simulink model "Par_model_sim_CHBjt9"  (R2023b)
settings: Solver=FixedStepAuto  StartTime=0.0  StopTime=5  FixedStep=1e-6  RelTol=1e-3
InitFcn:
  | sysinit
values from neighbouring files (symbols this model uses):
  C = 0.0234    [sysinit.m]
  f = 50    [sysinit.m]
  f_out = frequency_out_start : frequency_out_interval : frequency_out_end    [simout_chb_par.m]    (also in simout_chbjt_par.m = frequency_modulate_start : frequency_modulate_interval : fre)
  fn = 50    [sysinit.m]
  L = 0.002    [sysinit.m]
  L_ori = 0.02    [sysinit.m]
  L_sec = 0.06    [sysinit.m]
  m = 0.95    [sysinit.m]
  P0 = 8e6    (= 8000000)    [sysinit.m]
  R = 1.5    [sysinit.m]
  Source_Amp = 10000    [sysinit.m]
  st = 1e-6    (= 1e-06)    [sysinit.m]
  Td = 15e-7    (= 1.5e-06)    [sysinit.m]
  Ts2 = 0.5e-3    (= 0.0005)    [sysinit.m]
  U_dcN = 2500    [sysinit.m]
  Ul_in = 1900    [sysinit.m]
undefined symbols (not defined in the file or in its folder): magnitude
libraries: spsSeriesRLCBranchLib x123, spsDiodeLib x60, spsIGBTLib x48, spsMeanLib x20, spsCurrentMeasurementLib x16, spsThreePhaseVIMeasurementLib x13, spsOnDelayLib x12, spsUniversalBridgeLib x12, spsMultiWindingTransformerLib x9, simulink x5, spsRMSLib x4, spsVoltageMeasurementLib x3
(part 1 of 3)
settings Model: SimulationMode=accelerator  Creator=Jhchen  LastModifiedBy=Jhchen
settings DataIOCC: ReturnWorkspaceOutputs=off
settings DebuggingCC: RTPrefix=warning

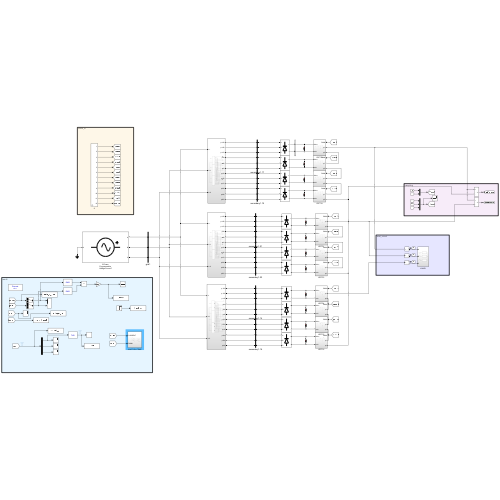
[thumbnail: Simulink's stored preview of the top-level diagram]
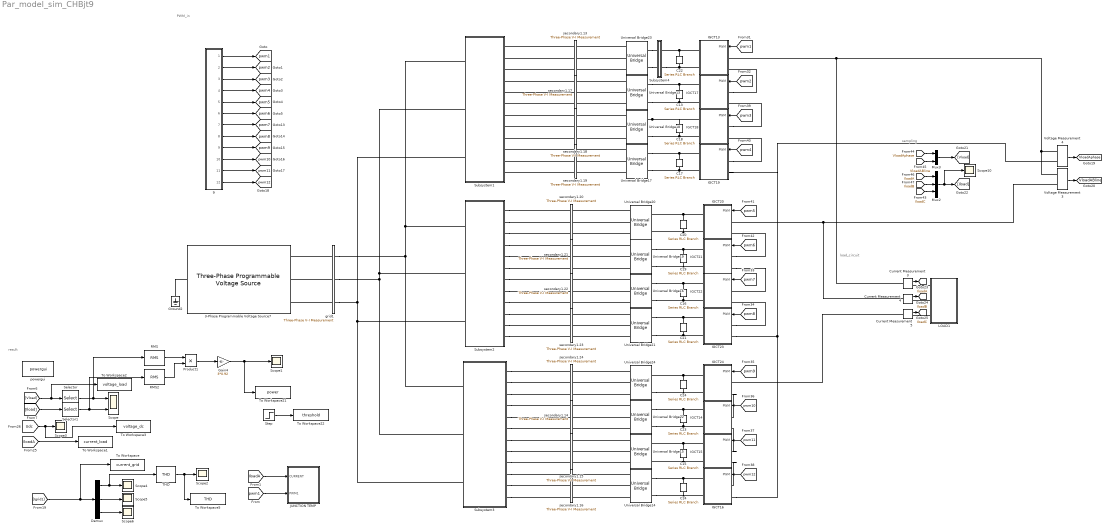
== system Par_model_sim_CHBjt9 ==
  note: PWM_in
  note: result
  note: load_circuit
  note: sampling
  3-Phase Programmable Voltage Source7 : spsThreePhaseProgrammableVoltageSourceLib/Three-Phase Programmable Voltage Source  PositiveSequence=[Source_Amp 0 fn]  VariationEntity=None  VariationType=Step  VariationTypeAlt=Step  VariationStep=0.5  VariationRate=10  VariationMagnitude=0.3  VariationFrequency=2  VariationTiming=[0.05 1]  VariationPhaseA=off  Amplitudes=[1 0.8 1.2 1.0]  TimeValues=[0 0.1 0.15 0.2]  HarmonicGeneration=off  HarmonicA=[5 0.08 -45 2]  HarmonicB=[2 0 0 2]  Timing="[0.1  1]"  BusType=swing  Pref=0  Qref=0  Qmin=-inf  Qmax=inf
  9 : Subsystem  mask{m=m, f=f, f_car=f_out, tt=1/8, ttd=Td}
      mask prompts: m "m_p"; f "f_module"; f_car "f_carrier"; tt "ts"; ttd "td"
      mask DialogControl ParameterGroupVar Prompt: 参数
  C{13..24} (12 alike) : spsSeriesRLCBranchLib/Series RLC Branch  LConnTagsString=__new0  RConnTagsString=__new0  BranchType=C  Resistance=0.0001  Inductance=1.0  SetiL0=off  InitialCurrent=0  Capacitance=C  Setx0=on  InitialVoltage=2500  Measurements=None
  Current Measurement3 : spsCurrentMeasurementLib/Current Measurement  PhasorSimulation=off  OutputType=Complex  PSBequivalent=0
  Current Measurement4 : spsCurrentMeasurementLib/Current Measurement  PhasorSimulation=off  OutputType=Complex  PSBequivalent=0
  Current Measurement5 : spsCurrentMeasurementLib/Current Measurement  PhasorSimulation=off  OutputType=Complex  PSBequivalent=0
  Demux : Demux  Outputs=3
  Gain4 : Gain  Gain=3*0.92
  Ground2 : spsGroundLib/Ground  LConnTagsString=a
  IGCT13 : Subsystem
      settings: PortSchema="{\"entries\":[{\"content\":{\"sides\":[{\"content\":{\"connectorIds\":[\"LConn1\",\"LConn2\"]},\"type\":\"ConnectorPlacement.EquallySpacedRectSide\",\"uuid\":\"3b5227fd-32cc-4097-9a6a-2909540651e9\"},{\"content\":{\"connectorIds\":[\"In1\",\"RConn1\",\"RConn2\"],\"side\":\"RIGHT\"},\"type\":\"ConnectorPlacement.EquallySpacedRectSide\",\"uuid\":\"b0068562-9d9a-456b-acd2-db870c5bcace\"},{\"content\":{\"side\":\"TOP\"},\"type\":\"ConnectorPlacement.EquallySpacedRectSide\",\"uuid\":\"bbecbe08-a8e7-4703-9f6f-443f87d924da\"}]},\"type\":\"ConnectorPlacement.EquallySpacedConnector\",\"uuid\":\"6ec83c7b-e3bb-4502-bc8f-4da9ff103a20\"}],\"packageUris\":[\"http://schema.mathworks.com/mf0/Connector/R2020b\"],\"version\":\"1.0\"}"
  IGCT14 : Subsystem
      settings: PortSchema="{\"entries\":[{\"content\":{\"sides\":[{\"content\":{\"connectorIds\":[\"LConn1\",\"LConn2\"]},\"type\":\"ConnectorPlacement.EquallySpacedRectSide\",\"uuid\":\"3b5227fd-32cc-4097-9a6a-2909540651e9\"},{\"content\":{\"connectorIds\":[\"In1\",\"RConn1\",\"RConn2\"],\"side\":\"RIGHT\"},\"type\":\"ConnectorPlacement.EquallySpacedRectSide\",\"uuid\":\"b0068562-9d9a-456b-acd2-db870c5bcace\"},{\"content\":{\"side\":\"TOP\"},\"type\":\"ConnectorPlacement.EquallySpacedRectSide\",\"uuid\":\"bbecbe08-a8e7-4703-9f6f-443f87d924da\"}]},\"type\":\"ConnectorPlacement.EquallySpacedConnector\",\"uuid\":\"6ec83c7b-e3bb-4502-bc8f-4da9ff103a20\"}],\"packageUris\":[\"http://schema.mathworks.com/mf0/Connector/R2020b\"],\"version\":\"1.0\"}"
  IGCT15 : Subsystem
      settings: PortSchema="{\"entries\":[{\"content\":{\"sides\":[{\"content\":{\"connectorIds\":[\"LConn1\",\"LConn2\"]},\"type\":\"ConnectorPlacement.EquallySpacedRectSide\",\"uuid\":\"3b5227fd-32cc-4097-9a6a-2909540651e9\"},{\"content\":{\"connectorIds\":[\"In1\",\"RConn1\",\"RConn2\"],\"side\":\"RIGHT\"},\"type\":\"ConnectorPlacement.EquallySpacedRectSide\",\"uuid\":\"b0068562-9d9a-456b-acd2-db870c5bcace\"},{\"content\":{\"side\":\"TOP\"},\"type\":\"ConnectorPlacement.EquallySpacedRectSide\",\"uuid\":\"bbecbe08-a8e7-4703-9f6f-443f87d924da\"}]},\"type\":\"ConnectorPlacement.EquallySpacedConnector\",\"uuid\":\"6ec83c7b-e3bb-4502-bc8f-4da9ff103a20\"}],\"packageUris\":[\"http://schema.mathworks.com/mf0/Connector/R2020b\"],\"version\":\"1.0\"}"
  IGCT16 : Subsystem
      settings: PortSchema="{\"entries\":[{\"content\":{\"sides\":[{\"content\":{\"connectorIds\":[\"LConn1\",\"LConn2\"]},\"type\":\"ConnectorPlacement.EquallySpacedRectSide\",\"uuid\":\"3b5227fd-32cc-4097-9a6a-2909540651e9\"},{\"content\":{\"connectorIds\":[\"In1\",\"RConn1\",\"RConn2\"],\"side\":\"RIGHT\"},\"type\":\"ConnectorPlacement.EquallySpacedRectSide\",\"uuid\":\"b0068562-9d9a-456b-acd2-db870c5bcace\"},{\"content\":{\"side\":\"TOP\"},\"type\":\"ConnectorPlacement.EquallySpacedRectSide\",\"uuid\":\"bbecbe08-a8e7-4703-9f6f-443f87d924da\"}]},\"type\":\"ConnectorPlacement.EquallySpacedConnector\",\"uuid\":\"6ec83c7b-e3bb-4502-bc8f-4da9ff103a20\"}],\"packageUris\":[\"http://schema.mathworks.com/mf0/Connector/R2020b\"],\"version\":\"1.0\"}"
  IGCT17 : Subsystem
      settings: PortSchema="{\"entries\":[{\"content\":{\"sides\":[{\"content\":{\"connectorIds\":[\"LConn1\",\"LConn2\"]},\"type\":\"ConnectorPlacement.EquallySpacedRectSide\",\"uuid\":\"3b5227fd-32cc-4097-9a6a-2909540651e9\"},{\"content\":{\"connectorIds\":[\"In1\",\"RConn1\",\"RConn2\"],\"side\":\"RIGHT\"},\"type\":\"ConnectorPlacement.EquallySpacedRectSide\",\"uuid\":\"b0068562-9d9a-456b-acd2-db870c5bcace\"},{\"content\":{\"side\":\"TOP\"},\"type\":\"ConnectorPlacement.EquallySpacedRectSide\",\"uuid\":\"bbecbe08-a8e7-4703-9f6f-443f87d924da\"}]},\"type\":\"ConnectorPlacement.EquallySpacedConnector\",\"uuid\":\"6ec83c7b-e3bb-4502-bc8f-4da9ff103a20\"}],\"packageUris\":[\"http://schema.mathworks.com/mf0/Connector/R2020b\"],\"version\":\"1.0\"}"
  IGCT18 : Subsystem
      settings: PortSchema="{\"entries\":[{\"content\":{\"sides\":[{\"content\":{\"connectorIds\":[\"LConn1\",\"LConn2\"]},\"type\":\"ConnectorPlacement.EquallySpacedRectSide\",\"uuid\":\"3b5227fd-32cc-4097-9a6a-2909540651e9\"},{\"content\":{\"connectorIds\":[\"In1\",\"RConn1\",\"RConn2\"],\"side\":\"RIGHT\"},\"type\":\"ConnectorPlacement.EquallySpacedRectSide\",\"uuid\":\"b0068562-9d9a-456b-acd2-db870c5bcace\"},{\"content\":{\"side\":\"TOP\"},\"type\":\"ConnectorPlacement.EquallySpacedRectSide\",\"uuid\":\"bbecbe08-a8e7-4703-9f6f-443f87d924da\"}]},\"type\":\"ConnectorPlacement.EquallySpacedConnector\",\"uuid\":\"6ec83c7b-e3bb-4502-bc8f-4da9ff103a20\"}],\"packageUris\":[\"http://schema.mathworks.com/mf0/Connector/R2020b\"],\"version\":\"1.0\"}"
  IGCT19 : Subsystem
      settings: PortSchema="{\"entries\":[{\"content\":{\"sides\":[{\"content\":{\"connectorIds\":[\"LConn1\",\"LConn2\"]},\"type\":\"ConnectorPlacement.EquallySpacedRectSide\",\"uuid\":\"3b5227fd-32cc-4097-9a6a-2909540651e9\"},{\"content\":{\"connectorIds\":[\"In1\",\"RConn1\",\"RConn2\"],\"side\":\"RIGHT\"},\"type\":\"ConnectorPlacement.EquallySpacedRectSide\",\"uuid\":\"b0068562-9d9a-456b-acd2-db870c5bcace\"},{\"content\":{\"side\":\"TOP\"},\"type\":\"ConnectorPlacement.EquallySpacedRectSide\",\"uuid\":\"bbecbe08-a8e7-4703-9f6f-443f87d924da\"}]},\"type\":\"ConnectorPlacement.EquallySpacedConnector\",\"uuid\":\"6ec83c7b-e3bb-4502-bc8f-4da9ff103a20\"}],\"packageUris\":[\"http://schema.mathworks.com/mf0/Connector/R2020b\"],\"version\":\"1.0\"}"
  IGCT20 : Subsystem
      settings: PortSchema="{\"entries\":[{\"content\":{\"sides\":[{\"content\":{\"connectorIds\":[\"LConn1\",\"LConn2\"]},\"type\":\"ConnectorPlacement.EquallySpacedRectSide\",\"uuid\":\"3b5227fd-32cc-4097-9a6a-2909540651e9\"},{\"content\":{\"connectorIds\":[\"In1\",\"RConn1\",\"RConn2\"],\"side\":\"RIGHT\"},\"type\":\"ConnectorPlacement.EquallySpacedRectSide\",\"uuid\":\"b0068562-9d9a-456b-acd2-db870c5bcace\"},{\"content\":{\"side\":\"TOP\"},\"type\":\"ConnectorPlacement.EquallySpacedRectSide\",\"uuid\":\"bbecbe08-a8e7-4703-9f6f-443f87d924da\"}]},\"type\":\"ConnectorPlacement.EquallySpacedConnector\",\"uuid\":\"6ec83c7b-e3bb-4502-bc8f-4da9ff103a20\"}],\"packageUris\":[\"http://schema.mathworks.com/mf0/Connector/R2020b\"],\"version\":\"1.0\"}"
  IGCT21 : Subsystem
      settings: PortSchema="{\"entries\":[{\"content\":{\"sides\":[{\"content\":{\"connectorIds\":[\"LConn1\",\"LConn2\"]},\"type\":\"ConnectorPlacement.EquallySpacedRectSide\",\"uuid\":\"3b5227fd-32cc-4097-9a6a-2909540651e9\"},{\"content\":{\"connectorIds\":[\"In1\",\"RConn1\",\"RConn2\"],\"side\":\"RIGHT\"},\"type\":\"ConnectorPlacement.EquallySpacedRectSide\",\"uuid\":\"b0068562-9d9a-456b-acd2-db870c5bcace\"},{\"content\":{\"side\":\"TOP\"},\"type\":\"ConnectorPlacement.EquallySpacedRectSide\",\"uuid\":\"bbecbe08-a8e7-4703-9f6f-443f87d924da\"}]},\"type\":\"ConnectorPlacement.EquallySpacedConnector\",\"uuid\":\"6ec83c7b-e3bb-4502-bc8f-4da9ff103a20\"}],\"packageUris\":[\"http://schema.mathworks.com/mf0/Connector/R2020b\"],\"version\":\"1.0\"}"
  IGCT22 : Subsystem
      settings: PortSchema="{\"entries\":[{\"content\":{\"sides\":[{\"content\":{\"connectorIds\":[\"LConn1\",\"LConn2\"]},\"type\":\"ConnectorPlacement.EquallySpacedRectSide\",\"uuid\":\"3b5227fd-32cc-4097-9a6a-2909540651e9\"},{\"content\":{\"connectorIds\":[\"In1\",\"RConn1\",\"RConn2\"],\"side\":\"RIGHT\"},\"type\":\"ConnectorPlacement.EquallySpacedRectSide\",\"uuid\":\"b0068562-9d9a-456b-acd2-db870c5bcace\"},{\"content\":{\"side\":\"TOP\"},\"type\":\"ConnectorPlacement.EquallySpacedRectSide\",\"uuid\":\"bbecbe08-a8e7-4703-9f6f-443f87d924da\"}]},\"type\":\"ConnectorPlacement.EquallySpacedConnector\",\"uuid\":\"6ec83c7b-e3bb-4502-bc8f-4da9ff103a20\"}],\"packageUris\":[\"http://schema.mathworks.com/mf0/Connector/R2020b\"],\"version\":\"1.0\"}"
  IGCT23 : Subsystem
      settings: PortSchema="{\"entries\":[{\"content\":{\"sides\":[{\"content\":{\"connectorIds\":[\"LConn1\",\"LConn2\"]},\"type\":\"ConnectorPlacement.EquallySpacedRectSide\",\"uuid\":\"3b5227fd-32cc-4097-9a6a-2909540651e9\"},{\"content\":{\"connectorIds\":[\"In1\",\"RConn1\",\"RConn2\"],\"side\":\"RIGHT\"},\"type\":\"ConnectorPlacement.EquallySpacedRectSide\",\"uuid\":\"b0068562-9d9a-456b-acd2-db870c5bcace\"},{\"content\":{\"side\":\"TOP\"},\"type\":\"ConnectorPlacement.EquallySpacedRectSide\",\"uuid\":\"bbecbe08-a8e7-4703-9f6f-443f87d924da\"}]},\"type\":\"ConnectorPlacement.EquallySpacedConnector\",\"uuid\":\"6ec83c7b-e3bb-4502-bc8f-4da9ff103a20\"}],\"packageUris\":[\"http://schema.mathworks.com/mf0/Connector/R2020b\"],\"version\":\"1.0\"}"
  IGCT24 : Subsystem
      settings: PortSchema="{\"entries\":[{\"content\":{\"sides\":[{\"content\":{\"connectorIds\":[\"LConn1\",\"LConn2\"]},\"type\":\"ConnectorPlacement.EquallySpacedRectSide\",\"uuid\":\"3b5227fd-32cc-4097-9a6a-2909540651e9\"},{\"content\":{\"connectorIds\":[\"In1\",\"RConn1\",\"RConn2\"],\"side\":\"RIGHT\"},\"type\":\"ConnectorPlacement.EquallySpacedRectSide\",\"uuid\":\"b0068562-9d9a-456b-acd2-db870c5bcace\"},{\"content\":{\"side\":\"TOP\"},\"type\":\"ConnectorPlacement.EquallySpacedRectSide\",\"uuid\":\"bbecbe08-a8e7-4703-9f6f-443f87d924da\"}]},\"type\":\"ConnectorPlacement.EquallySpacedConnector\",\"uuid\":\"6ec83c7b-e3bb-4502-bc8f-4da9ff103a20\"}],\"packageUris\":[\"http://schema.mathworks.com/mf0/Connector/R2020b\"],\"version\":\"1.0\"}"
  JUNCTION TEMP : Subsystem
  LOAD1 : Subsystem
  Mux2 : Mux  Inputs=3
  Mux3 : Mux  Inputs=2
  Product1 : Product
  RMS : spsRMSLib/RMS  TrueRMS=on  Freq=f  RMSInit=0  Ts=0
  RMS2 : spsRMSLib/RMS  TrueRMS=on  Freq=f  RMSInit=0  Ts=0
  Scope : Scope  NumInputPorts=2
  Scope{1..6,10} (7 alike) : Scope
  Selector : Selector  InputPortWidth=2  IndexOptions=Index vector (dialog)  Indices=[1]  OutputSizes=1
  Selector1 : Selector  InputPortWidth=3  IndexOptions=Index vector (dialog)  Indices=[1]  OutputSizes=1
  Step : Step  Time=0  Before=140  After=140  SampleTime=0
  Subsystem1 : Subsystem
  Subsystem2 : Subsystem
  Subsystem3 : Subsystem
  Subsystem4 : Subsystem
  THD : spsTHDLib/THD  Freq=f  Ts=0
  To Workspace : ToWorkspace  VariableName=current_grid  SaveFormat=Structure With Time  SampleTime=-1
  To Workspace1 : ToWorkspace  VariableName=current_load  SaveFormat=Structure With Time  SampleTime=-1
  To Workspace2 : ToWorkspace  VariableName=voltage_load  SaveFormat=Structure With Time  SampleTime=-1
  To Workspace21 : ToWorkspace  VariableName=power  SaveFormat=Structure With Time  SampleTime=-1
  To Workspace22 : ToWorkspace  VariableName=threshold  SaveFormat=Structure With Time  SampleTime=-1
  To Workspace3 : ToWorkspace  VariableName=voltage_dc  SaveFormat=Structure With Time  SampleTime=-1
  To Workspace5 : ToWorkspace  VariableName=THD  SaveFormat=Structure With Time  SampleTime=-1
  Universal Bridge{13..24} (12 alike) : spsUniversalBridgeLib/Universal Bridge  Arms=3  SnubberResistance=1e5  SnubberCapacitance=inf  Device=Diodes  Ron=1e-3  Lon=0  ForwardVoltages="[  0  0  ]"  ForwardVoltage=0  GTOparameters=[ 10e-6 , 20e-6 ]  IGBTparameters=[ 1e-6 , 2e-6 ]  Measurements=None  Measurements_2=None  converterType=Rectifier
  Voltage Measurement3 : spsVoltageMeasurementLib/Voltage Measurement  PhasorSimulation=off  OutputType=Complex  PSBequivalent=0
  Voltage Measurement4 : spsVoltageMeasurementLib/Voltage Measurement  PhasorSimulation=off  OutputType=Complex  PSBequivalent=0
  grid1 : spsThreePhaseVIMeasurementLib/Three-Phase V-I Measurement  VoltageMeasurement=phase-to-ground  SetLabelV=on  LabelV=Vgrid1  Vpu=off  VpuLL=off  CurrentMeasurement=yes  SetLabelI=on  LabelI=Igrid1  Ipu=off  Pbase=1e3  Vbase=380  OutputType=Magnitude  PhasorSimulation=off  PSBequivalent=0
  powergui : spspowerguiLib/powergui  Priority=1  SimulationMode=Discrete  SampleTime=st  frequency=60  Iterations=50  frequencyindice=50  Pbase=100e6  ErrMax=1e-4  UnitsV=kV  UnitsW=MW  buscounter=0  FunctionMessages=off  echomessages=off  EnableUseOfTLC=off  CurrentSourceSwitches=off  DisableSnubberDevices=off  DisableRonSwitches=off  DisableVfSwitches=off  DisplayEquations=off  AutomaticDiscreteSolvers=off  SolverType=Tustin/Backward Euler (TBE)  Interpol=off  ExternalGateDelay=off  methode=off  Ts=100  x0status=blocks  SPID=on  SwTol=0  HookPort=off  NonlinearTolerance=1e-4  nMaxIteration=100  ContinueOnMaxIteration=off  RestoreLinks=warning  ResistiveCurrentMeasurement=off  Frange=[0:2:500]  Ylog=off  Xlog=on  ShowGrid=off  save=off  variable=ZData  structure=0  ZoomFFT=off  StartTime=0.0  cycles=1  DisplayStyle=1  fundamental=60  FreqAxis=off  MaxFrequency=1000  frequencyindicesteady=1  RmsSteady=1  display=off
  secondary1.13 : spsThreePhaseVIMeasurementLib/Three-Phase V-I Measurement  VoltageMeasurement=phase-to-phase  SetLabelV=on  LabelV=Vsecondary_a1  Vpu=off  VpuLL=off  CurrentMeasurement=yes  SetLabelI=on  LabelI=Isecondary_a1  Ipu=off  Pbase=1e3  Vbase=380  OutputType=Magnitude  PhasorSimulation=off  PSBequivalent=0
  secondary1.14 : spsThreePhaseVIMeasurementLib/Three-Phase V-I Measurement  VoltageMeasurement=phase-to-phase  SetLabelV=on  LabelV=Vsecondary_c2  Vpu=off  VpuLL=off  CurrentMeasurement=yes  SetLabelI=on  LabelI=Isecondary_c2  Ipu=off  Pbase=1e3  Vbase=380  OutputType=Magnitude  PhasorSimulation=off  PSBequivalent=0
  secondary1.15 : spsThreePhaseVIMeasurementLib/Three-Phase V-I Measurement  VoltageMeasurement=phase-to-phase  SetLabelV=on  LabelV=Vsecondary_c3  Vpu=off  VpuLL=off  CurrentMeasurement=yes  SetLabelI=on  LabelI=Isecondary_c3  Ipu=off  Pbase=1e3  Vbase=380  OutputType=Magnitude  PhasorSimulation=off  PSBequivalent=0
  secondary1.16 : spsThreePhaseVIMeasurementLib/Three-Phase V-I Measurement  VoltageMeasurement=phase-to-phase  SetLabelV=on  LabelV=Vsecondary_c4  Vpu=off  VpuLL=off  CurrentMeasurement=yes  SetLabelI=on  LabelI=Isecondary_c4  Ipu=off  Pbase=1e3  Vbase=380  OutputType=Magnitude  PhasorSimulation=off  PSBequivalent=0
  secondary1.17 : spsThreePhaseVIMeasurementLib/Three-Phase V-I Measurement  VoltageMeasurement=phase-to-phase  SetLabelV=on  LabelV=Vsecondary_a2  Vpu=off  VpuLL=off  CurrentMeasurement=yes  SetLabelI=on  LabelI=Isecondary_a2  Ipu=off  Pbase=1e3  Vbase=380  OutputType=Magnitude  PhasorSimulation=off  PSBequivalent=0
  secondary1.18 : spsThreePhaseVIMeasurementLib/Three-Phase V-I Measurement  VoltageMeasurement=phase-to-phase  SetLabelV=on  LabelV=Vsecondary_a3  Vpu=off  VpuLL=off  CurrentMeasurement=yes  SetLabelI=on  LabelI=Isecondary_a3  Ipu=off  Pbase=1e3  Vbase=380  OutputType=Magnitude  PhasorSimulation=off  PSBequivalent=0
  secondary1.19 : spsThreePhaseVIMeasurementLib/Three-Phase V-I Measurement  VoltageMeasurement=phase-to-phase  SetLabelV=on  LabelV=Vsecondary_a4  Vpu=off  VpuLL=off  CurrentMeasurement=yes  SetLabelI=on  LabelI=Isecondary_a4  Ipu=off  Pbase=1e3  Vbase=380  OutputType=Magnitude  PhasorSimulation=off  PSBequivalent=0
  secondary1.20 : spsThreePhaseVIMeasurementLib/Three-Phase V-I Measurement  VoltageMeasurement=phase-to-phase  SetLabelV=on  LabelV=Vsecondary_b1  Vpu=off  VpuLL=off  CurrentMeasurement=yes  SetLabelI=on  LabelI=Isecondary_b1  Ipu=off  Pbase=1e3  Vbase=380  OutputType=Magnitude  PhasorSimulation=off  PSBequivalent=0
  secondary1.21 : spsThreePhaseVIMeasurementLib/Three-Phase V-I Measurement  VoltageMeasurement=phase-to-phase  SetLabelV=on  LabelV=Vsecondary_b2  Vpu=off  VpuLL=off  CurrentMeasurement=yes  SetLabelI=on  LabelI=Isecondary_b2  Ipu=off  Pbase=1e3  Vbase=380  OutputType=Magnitude  PhasorSimulation=off  PSBequivalent=0
  secondary1.22 : spsThreePhaseVIMeasurementLib/Three-Phase V-I Measurement  VoltageMeasurement=phase-to-phase  SetLabelV=on  LabelV=Vsecondary_b3  Vpu=off  VpuLL=off  CurrentMeasurement=yes  SetLabelI=on  LabelI=Isecondary_b3  Ipu=off  Pbase=1e3  Vbase=380  OutputType=Magnitude  PhasorSimulation=off  PSBequivalent=0
  secondary1.23 : spsThreePhaseVIMeasurementLib/Three-Phase V-I Measurement  VoltageMeasurement=phase-to-phase  SetLabelV=on  LabelV=Vsecondary_b4  Vpu=off  VpuLL=off  CurrentMeasurement=yes  SetLabelI=on  LabelI=Isecondary_b4  Ipu=off  Pbase=1e3  Vbase=380  OutputType=Magnitude  PhasorSimulation=off  PSBequivalent=0
  secondary1.24 : spsThreePhaseVIMeasurementLib/Three-Phase V-I Measurement  VoltageMeasurement=phase-to-phase  SetLabelV=on  LabelV=Vsecondary_c1  Vpu=off  VpuLL=off  CurrentMeasurement=yes  SetLabelI=on  LabelI=Isecondary_c1  Ipu=off  Pbase=1e3  Vbase=380  OutputType=Magnitude  PhasorSimulation=off  PSBequivalent=0
  tag scope: IloadA=global, IloadB=global, IloadC=global, VloadABline=global, VloadAphase=global, pwm10=global, pwm11=global, pwm12=global, pwm1=global, pwm2=global, pwm3=global, pwm4=global, pwm5=global, pwm6=global, pwm7=global, pwm8=global, pwm9=global
  wires:
  Selector/1 -> Scope/1, RMS/1
  Selector1/1 -> RMS2/1, Scope/2
  [IloadA] -> To Workspace1/1
  [Udc] -> To Workspace3/1, Scope3/1
  9/1(Output) -> [pwm1]
  9/2(Output1) -> [pwm2]
  9/3(Output2) -> [pwm3]
  9/4(Output3) -> [pwm4]
  9/5(Output4) -> [pwm5]
  9/6(Output5) -> [pwm6]
  9/7(Output6) -> [pwm7]
  9/8(Output7) -> [pwm8]
  9/9(Output8) -> [pwm9]
  9/10(Output9) -> [pwm10]
  9/11(Output10) -> [pwm11]
  9/12(Output11) -> [pwm12]
  [Igrid1] -> Demux/1, To Workspace/1
  Demux/1 -> THD/1, Scope4/1
  Demux/2 -> Scope5/1
  Demux/3 -> Scope6/1
  [pwm7] -> IGCT22/1(PWM)
  [pwm8] -> IGCT23/1(PWM)
  [pwm9] -> IGCT24/1(PWM)
  [pwm10] -> IGCT14/1(PWM)
  [pwm11] -> IGCT15/1(PWM)
  [pwm12] -> IGCT16/1(PWM)
  [pwm6] -> IGCT21/1(PWM)
  [pwm5] -> IGCT20/1(PWM)
  [pwm4] -> IGCT19/1(PWM)
  [pwm3] -> IGCT18/1(PWM)
  [pwm2] -> IGCT17/1(PWM)
  [pwm1] -> IGCT13/1(PWM)
  Mux3/1 -> [Vload]
  [VloadAphase] -> Mux3/1
  Current Measurement3/1 -> [IloadA]
  [IloadB] -> Mux2/2
  Voltage Measurement3/1 -> [VloadABline]
  Mux2/1 -> Scope10/1, [Iload]
  Current Measurement4/1 -> [IloadB]
  Current Measurement5/1 -> [IloadC]
  [IloadC] -> Mux2/3
  [IloadA] -> Mux2/1
  [VloadABline] -> Mux3/2
  Voltage Measurement4/1 -> [VloadAphase]
  THD/1 -> Scope2/1, To Workspace5/1
  [Vload] -> To Workspace2/1, Selector/1
  Step/1 -> To Workspace22/1
  RMS/1 -> Product1/1
  RMS2/1 -> Product1/2
  Gain4/1 -> Scope1/1, To Workspace21/1
  Product1/1 -> Gain4/1
  [Iload] -> Selector1/1
  [pwm1] -> JUNCTION TEMP/2(PWM1)
  [IloadA] -> JUNCTION TEMP/1(CURRENT)
  connections:
  3-Phase Programmable Voltage Source7/LConn1 -- Ground2/LConn1
  Subsystem3/RConn8 -- secondary1.15/LConn2
  Universal Bridge21/LConn1 -- secondary1.23/RConn1
  Universal Bridge14/LConn2 -- secondary1.16/RConn2
  Universal Bridge15/LConn2 -- secondary1.15/RConn2
  Subsystem2/RConn11 -- secondary1.23/LConn2
  Universal Bridge16/LConn2 -- secondary1.22/RConn2
  Subsystem3/RConn9 -- secondary1.15/LConn3
  Subsystem2/RConn12 -- secondary1.23/LConn3
  Universal Bridge24/LConn1 -- secondary1.24/RConn1
  Universal Bridge16/LConn1 -- secondary1.22/RConn1
  Subsystem2/RConn9 -- secondary1.22/LConn3
  Subsystem2/RConn8 -- secondary1.22/LConn2
  Universal Bridge21/LConn2 -- secondary1.23/RConn2
  Universal Bridge16/LConn3 -- secondary1.22/RConn3
  Universal Bridge22/LConn1 -- secondary1.14/RConn1
  Subsystem2/RConn7 -- secondary1.22/LConn1
  Universal Bridge15/LConn1 -- secondary1.15/RConn1
  Universal Bridge22/LConn2 -- secondary1.14/RConn2
  Subsystem3/RConn2 -- secondary1.24/LConn2
  Subsystem3/RConn6 -- secondary1.14/LConn3
  Universal Bridge24/LConn2 -- secondary1.24/RConn2
  Subsystem3/RConn11 -- secondary1.16/LConn2
  Subsystem3/RConn7 -- secondary1.15/LConn1
  Subsystem3/RConn12 -- secondary1.16/LConn3
  Universal Bridge14/LConn1 -- secondary1.16/RConn1
  Universal Bridge15/LConn3 -- secondary1.15/RConn3
  Subsystem3/RConn10 -- secondary1.16/LConn1
  Subsystem2/RConn4 -- secondary1.21/LConn1
  Universal Bridge20/LConn1 -- secondary1.20/RConn1
  Universal Bridge19/LConn3 -- secondary1.21/RConn3
  Universal Bridge19/LConn1 -- secondary1.21/RConn1
  Subsystem2/RConn3 -- secondary1.20/LConn3
  Universal Bridge20/LConn2 -- secondary1.20/RConn2
  Subsystem2/RConn5 -- secondary1.21/LConn2
  Universal Bridge14/LConn3 -- secondary1.16/RConn3
  Subsystem2/RConn10 -- secondary1.23/LConn1
  Universal Bridge18/LConn2 -- secondary1.18/RConn2
  Subsystem3/RConn4 -- secondary1.14/LConn1
  secondary1.18/LConn1 -- Subsystem1/RConn7
  secondary1.19/LConn3 -- Subsystem1/RConn12
  Universal Bridge22/LConn3 -- secondary1.14/RConn3
  secondary1.18/LConn2 -- Subsystem1/RConn8
  Universal Bridge21/LConn3 -- secondary1.23/RConn3
  secondary1.19/LConn2 -- Subsystem1/RConn11
  Subsystem2/RConn1 -- secondary1.20/LConn1
  secondary1.19/LConn1 -- Subsystem1/RConn10
  Subsystem2/RConn6 -- secondary1.21/LConn3
  secondary1.18/LConn3 -- Subsystem1/RConn9
  Universal Bridge17/LConn1 -- secondary1.19/RConn1
  Universal Bridge19/LConn2 -- secondary1.21/RConn2
  Universal Bridge17/LConn2 -- secondary1.19/RConn2
  Subsystem3/RConn5 -- secondary1.14/LConn2
  Subsystem3/RConn3 -- secondary1.24/LConn3
  Universal Bridge18/LConn1 -- secondary1.18/RConn1
  Universal Bridge24/LConn3 -- secondary1.24/RConn3
  secondary1.13/LConn1 -- Subsystem1/RConn1
  Universal Bridge23/LConn1 -- secondary1.13/RConn1
  Universal Bridge13/LConn2 -- secondary1.17/RConn2
  Universal Bridge17/LConn3 -- secondary1.19/RConn3
  Universal Bridge23/LConn3 -- secondary1.13/RConn3
  Universal Bridge13/LConn3 -- secondary1.17/RConn3
  Universal Bridge13/LConn1 -- secondary1.17/RConn1
  Subsystem3/RConn1 -- secondary1.24/LConn1
  secondary1.13/LConn3 -- Subsystem1/RConn3
  secondary1.17/LConn1 -- Subsystem1/RConn4
  secondary1.13/LConn2 -- Subsystem1/RConn2
  secondary1.17/LConn3 -- Subsystem1/RConn6
  Universal Bridge23/LConn2 -- secondary1.13/RConn2
  Universal Bridge20/LConn3 -- secondary1.20/RConn3
  Universal Bridge18/LConn3 -- secondary1.18/RConn3
  secondary1.17/LConn2 -- Subsystem1/RConn5
  Subsystem2/RConn2 -- secondary1.20/LConn2
  Universal Bridge13/RConn2 -- IGCT17/LConn2 -- C13/RConn1
  Universal Bridge13/RConn1 -- IGCT17/LConn1 -- C13/LConn1
  Subsystem4/RConn2 -- IGCT13/LConn2 -- C22/RConn1
  C22/LConn1 -- IGCT13/LConn1 -- Subsystem4/RConn1
  Universal Bridge17/RConn2 -- IGCT19/LConn2 -- C17/RConn1
  Universal Bridge17/RConn1 -- IGCT19/LConn1 -- C17/LConn1
  Universal Bridge18/RConn2 -- IGCT18/LConn2 -- C18/RConn1
  Universal Bridge18/RConn1 -- C18/LConn1 -- IGCT18/LConn1
  C19/RConn1 -- Universal Bridge19/RConn2 -- IGCT21/LConn2
  C19/LConn1 -- Universal Bridge19/RConn1 -- IGCT21/LConn1
  C20/LConn1 -- IGCT20/LConn1 -- Universal Bridge20/RConn1
  C20/RConn1 -- IGCT20/LConn2 -- Universal Bridge20/RConn2
  Universal Bridge21/RConn2 -- IGCT23/LConn2 -- C21/RConn1
  Universal Bridge21/RConn1 -- IGCT23/LConn1 -- C21/LConn1
  Universal Bridge16/RConn2 -- IGCT22/LConn2 -- C16/RConn1
  C16/LConn1 -- Universal Bridge16/RConn1 -- IGCT22/LConn1
  Universal Bridge22/RConn2 -- IGCT14/LConn2 -- C23/RConn1
  Universal Bridge22/RConn1 -- IGCT14/LConn1 -- C23/LConn1
  C24/RConn1 -- Universal Bridge24/RConn2 -- IGCT24/LConn2
  C24/LConn1 -- IGCT24/LConn1 -- Universal Bridge24/RConn1
  C14/RConn1 -- Universal Bridge14/RConn2 -- IGCT16/LConn2
  C14/LConn1 -- Universal Bridge14/RConn1 -- IGCT16/LConn1
  C15/LConn1 -- IGCT15/LConn1 -- Universal Bridge15/RConn1
  C15/RConn1 -- IGCT15/LConn2 -- Universal Bridge15/RConn2
  IGCT16/RConn2 -- IGCT23/RConn2 -- Voltage Measurement4/LConn2 -- IGCT19/RConn2
  IGCT15/RConn1 -- IGCT14/RConn2
  IGCT24/RConn2 -- IGCT14/RConn1
  IGCT23/RConn1 -- IGCT22/RConn2
  IGCT15/RConn2 -- IGCT16/RConn1
  IGCT21/RConn2 -- IGCT22/RConn1
  IGCT21/RConn1 -- IGCT20/RConn2
  IGCT18/RConn1 -- IGCT17/RConn2
  IGCT19/RConn1 -- IGCT18/RConn2
  Universal Bridge23/RConn2 -- Subsystem4/LConn2
  Universal Bridge23/RConn1 -- Subsystem4/LConn1
  IGCT17/RConn1 -- IGCT13/RConn2
  Current Measurement5/LConn1 -- IGCT24/RConn1
  Voltage Measurement4/LConn1 -- Voltage Measurement3/LConn1 -- Current Measurement3/LConn1 -- IGCT13/RConn1
  Voltage Measurement3/LConn2 -- Current Measurement4/LConn1 -- IGCT20/RConn1
  Current Measurement3/RConn1 -- LOAD1/LConn1
  Current Measurement5/RConn1 -- LOAD1/LConn3
  LOAD1/LConn2 -- Current Measurement4/RConn1
  grid1/LConn3 -- 3-Phase Programmable Voltage Source7/RConn3
  grid1/LConn2 -- 3-Phase Programmable Voltage Source7/RConn2
  grid1/LConn1 -- 3-Phase Programmable Voltage Source7/RConn1
  grid1/RConn2 -- Subsystem2/LConn2 -- Subsystem1/LConn2 -- Subsystem3/LConn2
  grid1/RConn1 -- Subsystem2/LConn1 -- Subsystem1/LConn1 -- Subsystem3/LConn1
  grid1/RConn3 -- Subsystem3/LConn3 -- Subsystem2/LConn3 -- Subsystem1/LConn3

== system Par_model_sim_CHBjt9/9 ==
  -2/3*pi : Subsystem
  0 : Subsystem
  2/3*pi : Subsystem
  Sine Wave : Sin  Amplitude=m*1000  Frequency=f*2*pi  Phase=2/3*pi  SampleTime=0
  Sine Wave1 : Sin  Amplitude=m*1000  Frequency=f*2*pi  SampleTime=0
  Sine Wave2 : Sin  Amplitude=m*1000  Frequency=f*2*pi  Phase=-2/3*pi  SampleTime=0
  Subsystem : Subsystem
  Output : Outport
  Output1 : Outport  Port=2
  Output2 : Outport  Port=3
  Output3 : Outport  Port=4
  Output4 : Outport  Port=5
  Output5 : Outport  Port=6
  Output6 : Outport  Port=7
  Output7 : Outport  Port=8
  Output8 : Outport  Port=9
  Output9 : Outport  Port=10
  Output10 : Outport  Port=11
  Output11 : Outport  Port=12
  wires:
  Subsystem/3(Out3) -> -2/3*pi/1(In1)
  Subsystem/2(Out2) -> 0/1(In1)
  Subsystem/1(Out1) -> 2/3*pi/1(In1)
  Sine Wave2/1 -> Subsystem/3(In3)
  Sine Wave1/1 -> Subsystem/2(In2)
  Sine Wave/1 -> Subsystem/1(In1)
  2/3*pi/1(Output) -> Output/1
  0/1(Out1) -> Output4/1
  -2/3*pi/1(Output8) -> Output8/1
  -2/3*pi/2(Output9) -> Output9/1
  -2/3*pi/3(Output10) -> Output10/1
  -2/3*pi/4(Output11) -> Output11/1
  0/2(Output5) -> Output5/1
  0/3(Output6) -> Output6/1
  0/4(Output7) -> Output7/1
  2/3*pi/2(Output1) -> Output1/1
  2/3*pi/3(Output2) -> Output2/1
  2/3*pi/4(Output3) -> Output3/1

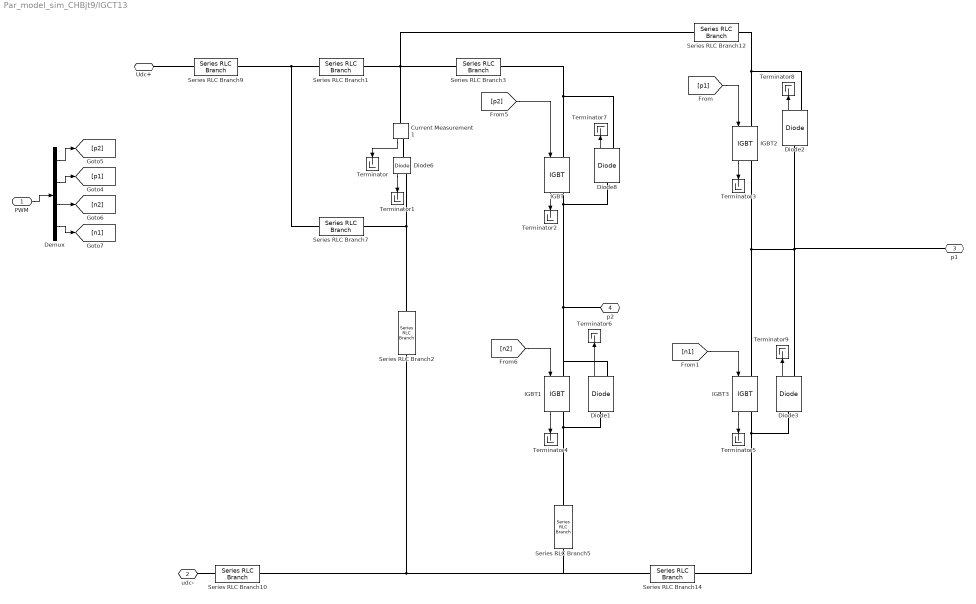
== system Par_model_sim_CHBjt9/IGCT13 ==
  PWM : Inport
  Current Measurement1 : spsCurrentMeasurementLib/Current Measurement  PhasorSimulation=off  OutputType=Complex  PSBequivalent=0
  Demux : Demux
  Diode{1..3,6,8} (5 alike) : spsDiodeLib/Diode  Ron=rto  Lon=0  Vf=vto  IC=0  UseSnubber=off  Rs=500  Cs=250e-9  Measurements=on
  IGBT{,1..3} (4 alike) : spsIGBTLib/IGBT  Ron=rt  Lon=0  Vf=vt  Tf=1e-6  Tt=2e-6  IC=0  Rs=1e5  Cs=inf  Measurements=on
  Series RLC Branch1 : spsSeriesRLCBranchLib/Series RLC Branch  LConnTagsString=__new0  RConnTagsString=__new0  BranchType=RL  Resistance=1e-5  Inductance=3.0E-6  SetiL0=off  InitialCurrent=0  Capacitance=1e-6  Setx0=off  InitialVoltage=0  Measurements=None
  Series RLC Branch10 : spsSeriesRLCBranchLib/Series RLC Branch  LConnTagsString=__new0  RConnTagsString=__new0  BranchType=L  Resistance=1  Inductance=0.4e-6  SetiL0=off  InitialCurrent=0  Capacitance=1e-6  Setx0=off  InitialVoltage=0  Measurements=None
  Series RLC Branch12 : spsSeriesRLCBranchLib/Series RLC Branch  LConnTagsString=__new0  RConnTagsString=__new0  BranchType=RL  Resistance=1e-5  Inductance=1E-9  SetiL0=off  InitialCurrent=0  Capacitance=1e-6  Setx0=off  InitialVoltage=0  Measurements=None
  Series RLC Branch14 : spsSeriesRLCBranchLib/Series RLC Branch  LConnTagsString=__new0  RConnTagsString=__new0  BranchType=L  Resistance=1  Inductance=1E-7  SetiL0=off  InitialCurrent=0  Capacitance=1e-6  Setx0=off  InitialVoltage=0  Measurements=None
  Series RLC Branch2 : spsSeriesRLCBranchLib/Series RLC Branch  LConnTagsString=__new0  RConnTagsString=__new0  BranchType=RC  Resistance=1e-5  Inductance=20e-6  SetiL0=off  InitialCurrent=0  Capacitance=17e-6  Setx0=off  InitialVoltage=0  Measurements=None
  Series RLC Branch3 : spsSeriesRLCBranchLib/Series RLC Branch  LConnTagsString=__new0  RConnTagsString=__new0  BranchType=RL  Resistance=1e-5  Inductance=1E-9  SetiL0=off  InitialCurrent=0  Capacitance=1e-6  Setx0=off  InitialVoltage=0  Measurements=None
  Series RLC Branch5 : spsSeriesRLCBranchLib/Series RLC Branch  LConnTagsString=__new0  RConnTagsString=__new0  BranchType=L  Resistance=1  Inductance=1E-7  SetiL0=off  InitialCurrent=0  Capacitance=1e-6  Setx0=off  InitialVoltage=0  Measurements=None
  Series RLC Branch7 : spsSeriesRLCBranchLib/Series RLC Branch  LConnTagsString=__new0  RConnTagsString=__new0  BranchType=RL  Resistance=0.6  Inductance=1e-6  SetiL0=off  InitialCurrent=0  Capacitance=1e-6  Setx0=off  InitialVoltage=0  Measurements=None
  Series RLC Branch9 : spsSeriesRLCBranchLib/Series RLC Branch  LConnTagsString=__new0  RConnTagsString=__new0  BranchType=L  Resistance=1  Inductance=0.4e-6  SetiL0=off  InitialCurrent=0  Capacitance=1e-6  Setx0=off  InitialVoltage=0  Measurements=None
  Terminator{,1..9} (10 alike) : Terminator
  Udc+ : PMIOPort  Side=Left
  udc- : PMIOPort  Port=2  Side=Left
  p1 : PMIOPort  Port=3  Side=Right
  p2 : PMIOPort  Port=4  Side=Right
  wires:
  Demux/4 -> [n1]
  Demux/2 -> [p1]
  Demux/1 -> [p2]
  PWM/1 -> Demux/1
  Demux/3 -> [n2]
  Diode6/1 -> Terminator1/1
  Diode1/1 -> Terminator6/1
  Diode8/1 -> Terminator7/1
  [p2] -> IGBT/1
  Diode2/1 -> Terminator8/1
  Current Measurement1/1 -> Terminator/1
  [p1] -> IGBT2/1
  [n2] -> IGBT1/1
  IGBT/1 -> Terminator2/1
  IGBT2/1 -> Terminator3/1
  IGBT1/1 -> Terminator4/1
  [n1] -> IGBT3/1
  IGBT3/1 -> Terminator5/1
  Diode3/1 -> Terminator9/1
  connections:
  IGBT/RConn1 -- Diode8/LConn1 -- Diode1/RConn1 -- IGBT1/LConn1 -- p2/RConn1
  Series RLC Branch9/RConn1 -- Series RLC Branch7/LConn1 -- Series RLC Branch1/LConn1
  Series RLC Branch2/RConn1 -- Series RLC Branch10/RConn1 -- Series RLC Branch14/LConn1 -- Series RLC Branch5/LConn1
  IGBT2/RConn1 -- IGBT3/LConn1 -- Diode3/RConn1 -- Diode2/LConn1 -- p1/RConn1
  IGBT2/LConn1 -- Series RLC Branch12/RConn1 -- Diode2/RConn1
  Current Measurement1/RConn1 -- Diode6/LConn1
  IGBT1/RConn1 -- Series RLC Branch5/RConn1 -- Diode1/LConn1
  Diode8/RConn1 -- IGBT/LConn1 -- Series RLC Branch3/RConn1
  Series RLC Branch14/RConn1 -- IGBT3/RConn1 -- Diode3/LConn1
  Series RLC Branch12/LConn1 -- Series RLC Branch3/LConn1 -- Series RLC Branch1/RConn1 -- Current Measurement1/LConn1
  Series RLC Branch2/LConn1 -- Series RLC Branch7/RConn1 -- Diode6/RConn1
  Series RLC Branch9/LConn1 -- Udc+/RConn1
  Series RLC Branch10/LConn1 -- udc-/RConn1

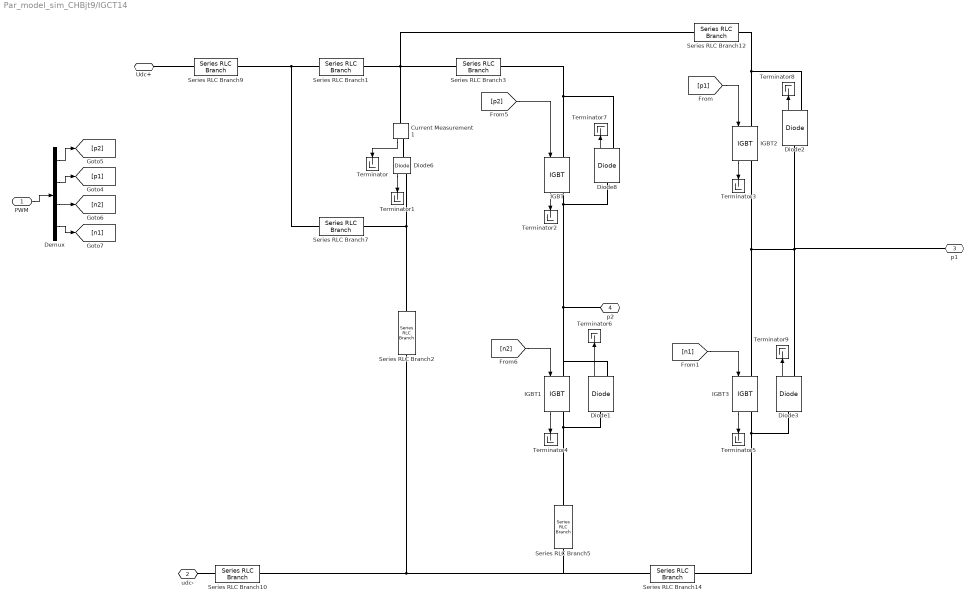
== system Par_model_sim_CHBjt9/IGCT14 ==
  PWM : Inport
  Current Measurement1 : spsCurrentMeasurementLib/Current Measurement  PhasorSimulation=off  OutputType=Complex  PSBequivalent=0
  Demux : Demux
  Diode{1..3,6,8} (5 alike) : spsDiodeLib/Diode  Ron=rto  Lon=0  Vf=vto  IC=0  UseSnubber=off  Rs=500  Cs=250e-9  Measurements=on
  IGBT{,1..3} (4 alike) : spsIGBTLib/IGBT  Ron=rt  Lon=0  Vf=vt  Tf=1e-6  Tt=2e-6  IC=0  Rs=1e5  Cs=inf  Measurements=on
  Series RLC Branch1 : spsSeriesRLCBranchLib/Series RLC Branch  LConnTagsString=__new0  RConnTagsString=__new0  BranchType=RL  Resistance=1e-5  Inductance=3.0E-6  SetiL0=off  InitialCurrent=0  Capacitance=1e-6  Setx0=off  InitialVoltage=0  Measurements=None
  Series RLC Branch10 : spsSeriesRLCBranchLib/Series RLC Branch  LConnTagsString=__new0  RConnTagsString=__new0  BranchType=L  Resistance=1  Inductance=0.4e-6  SetiL0=off  InitialCurrent=0  Capacitance=1e-6  Setx0=off  InitialVoltage=0  Measurements=None
  Series RLC Branch12 : spsSeriesRLCBranchLib/Series RLC Branch  LConnTagsString=__new0  RConnTagsString=__new0  BranchType=RL  Resistance=1e-5  Inductance=1E-9  SetiL0=off  InitialCurrent=0  Capacitance=1e-6  Setx0=off  InitialVoltage=0  Measurements=None
  Series RLC Branch14 : spsSeriesRLCBranchLib/Series RLC Branch  LConnTagsString=__new0  RConnTagsString=__new0  BranchType=L  Resistance=1  Inductance=1E-7  SetiL0=off  InitialCurrent=0  Capacitance=1e-6  Setx0=off  InitialVoltage=0  Measurements=None
  Series RLC Branch2 : spsSeriesRLCBranchLib/Series RLC Branch  LConnTagsString=__new0  RConnTagsString=__new0  BranchType=RC  Resistance=1e-5  Inductance=20e-6  SetiL0=off  InitialCurrent=0  Capacitance=17e-6  Setx0=off  InitialVoltage=0  Measurements=None
  Series RLC Branch3 : spsSeriesRLCBranchLib/Series RLC Branch  LConnTagsString=__new0  RConnTagsString=__new0  BranchType=RL  Resistance=1e-5  Inductance=1E-9  SetiL0=off  InitialCurrent=0  Capacitance=1e-6  Setx0=off  InitialVoltage=0  Measurements=None
  Series RLC Branch5 : spsSeriesRLCBranchLib/Series RLC Branch  LConnTagsString=__new0  RConnTagsString=__new0  BranchType=L  Resistance=1  Inductance=1E-7  SetiL0=off  InitialCurrent=0  Capacitance=1e-6  Setx0=off  InitialVoltage=0  Measurements=None
  Series RLC Branch7 : spsSeriesRLCBranchLib/Series RLC Branch  LConnTagsString=__new0  RConnTagsString=__new0  BranchType=RL  Resistance=0.6  Inductance=1e-6  SetiL0=off  InitialCurrent=0  Capacitance=1e-6  Setx0=off  InitialVoltage=0  Measurements=None
  Series RLC Branch9 : spsSeriesRLCBranchLib/Series RLC Branch  LConnTagsString=__new0  RConnTagsString=__new0  BranchType=L  Resistance=1  Inductance=0.4e-6  SetiL0=off  InitialCurrent=0  Capacitance=1e-6  Setx0=off  InitialVoltage=0  Measurements=None
  Terminator{,1..9} (10 alike) : Terminator
  Udc+ : PMIOPort  Side=Left
  udc- : PMIOPort  Port=2  Side=Left
  p1 : PMIOPort  Port=3  Side=Right
  p2 : PMIOPort  Port=4  Side=Right
  wires:
  Demux/4 -> [n1]
  Demux/2 -> [p1]
  Demux/1 -> [p2]
  PWM/1 -> Demux/1
  Demux/3 -> [n2]
  Diode6/1 -> Terminator1/1
  Diode1/1 -> Terminator6/1
  Diode8/1 -> Terminator7/1
  [p2] -> IGBT/1
  Diode2/1 -> Terminator8/1
  Current Measurement1/1 -> Terminator/1
  [p1] -> IGBT2/1
  [n2] -> IGBT1/1
  IGBT/1 -> Terminator2/1
  IGBT2/1 -> Terminator3/1
  IGBT1/1 -> Terminator4/1
  [n1] -> IGBT3/1
  IGBT3/1 -> Terminator5/1
  Diode3/1 -> Terminator9/1
  connections:
  IGBT/RConn1 -- Diode8/LConn1 -- Diode1/RConn1 -- IGBT1/LConn1 -- p2/RConn1
  Series RLC Branch9/RConn1 -- Series RLC Branch7/LConn1 -- Series RLC Branch1/LConn1
  Series RLC Branch2/RConn1 -- Series RLC Branch10/RConn1 -- Series RLC Branch14/LConn1 -- Series RLC Branch5/LConn1
  IGBT2/RConn1 -- IGBT3/LConn1 -- Diode3/RConn1 -- Diode2/LConn1 -- p1/RConn1
  IGBT2/LConn1 -- Series RLC Branch12/RConn1 -- Diode2/RConn1
  Current Measurement1/RConn1 -- Diode6/LConn1
  IGBT1/RConn1 -- Series RLC Branch5/RConn1 -- Diode1/LConn1
  Diode8/RConn1 -- IGBT/LConn1 -- Series RLC Branch3/RConn1
  Series RLC Branch14/RConn1 -- IGBT3/RConn1 -- Diode3/LConn1
  Series RLC Branch12/LConn1 -- Series RLC Branch3/LConn1 -- Series RLC Branch1/RConn1 -- Current Measurement1/LConn1
  Series RLC Branch2/LConn1 -- Series RLC Branch7/RConn1 -- Diode6/RConn1
  Series RLC Branch9/LConn1 -- Udc+/RConn1
  Series RLC Branch10/LConn1 -- udc-/RConn1

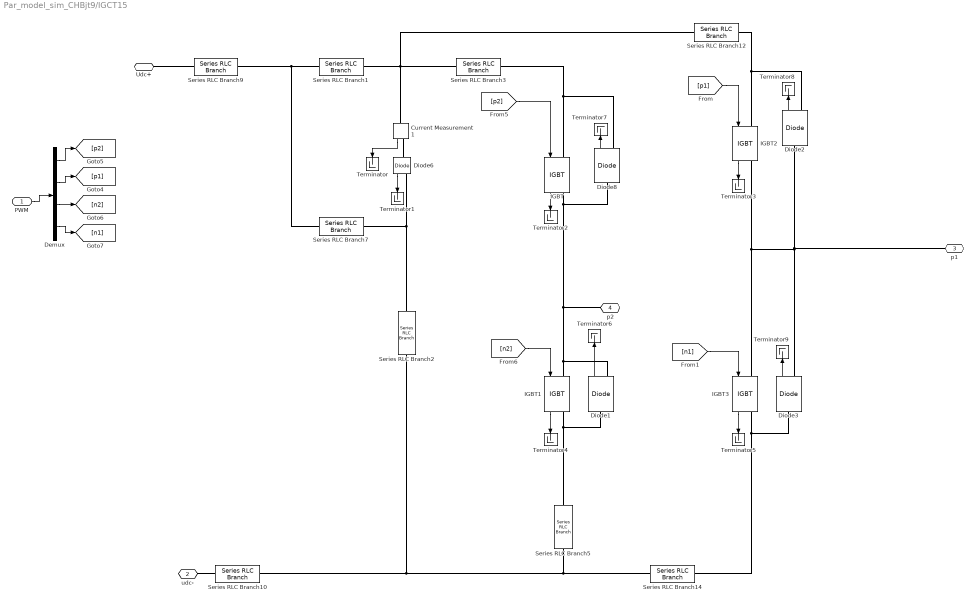
== system Par_model_sim_CHBjt9/IGCT15 ==
  PWM : Inport
  Current Measurement1 : spsCurrentMeasurementLib/Current Measurement  PhasorSimulation=off  OutputType=Complex  PSBequivalent=0
  Demux : Demux
  Diode{1..3,6,8} (5 alike) : spsDiodeLib/Diode  Ron=rto  Lon=0  Vf=vto  IC=0  UseSnubber=off  Rs=500  Cs=250e-9  Measurements=on
  IGBT{,1..3} (4 alike) : spsIGBTLib/IGBT  Ron=rt  Lon=0  Vf=vt  Tf=1e-6  Tt=2e-6  IC=0  Rs=1e5  Cs=inf  Measurements=on
  Series RLC Branch1 : spsSeriesRLCBranchLib/Series RLC Branch  LConnTagsString=__new0  RConnTagsString=__new0  BranchType=RL  Resistance=1e-5  Inductance=3.0E-6  SetiL0=off  InitialCurrent=0  Capacitance=1e-6  Setx0=off  InitialVoltage=0  Measurements=None
  Series RLC Branch10 : spsSeriesRLCBranchLib/Series RLC Branch  LConnTagsString=__new0  RConnTagsString=__new0  BranchType=L  Resistance=1  Inductance=0.4e-6  SetiL0=off  InitialCurrent=0  Capacitance=1e-6  Setx0=off  InitialVoltage=0  Measurements=None
  Series RLC Branch12 : spsSeriesRLCBranchLib/Series RLC Branch  LConnTagsString=__new0  RConnTagsString=__new0  BranchType=RL  Resistance=1e-5  Inductance=1E-9  SetiL0=off  InitialCurrent=0  Capacitance=1e-6  Setx0=off  InitialVoltage=0  Measurements=None
  Series RLC Branch14 : spsSeriesRLCBranchLib/Series RLC Branch  LConnTagsString=__new0  RConnTagsString=__new0  BranchType=L  Resistance=1  Inductance=1E-7  SetiL0=off  InitialCurrent=0  Capacitance=1e-6  Setx0=off  InitialVoltage=0  Measurements=None
  Series RLC Branch2 : spsSeriesRLCBranchLib/Series RLC Branch  LConnTagsString=__new0  RConnTagsString=__new0  BranchType=RC  Resistance=1e-5  Inductance=20e-6  SetiL0=off  InitialCurrent=0  Capacitance=17e-6  Setx0=off  InitialVoltage=0  Measurements=None
  Series RLC Branch3 : spsSeriesRLCBranchLib/Series RLC Branch  LConnTagsString=__new0  RConnTagsString=__new0  BranchType=RL  Resistance=1e-5  Inductance=1E-9  SetiL0=off  InitialCurrent=0  Capacitance=1e-6  Setx0=off  InitialVoltage=0  Measurements=None
  Series RLC Branch5 : spsSeriesRLCBranchLib/Series RLC Branch  LConnTagsString=__new0  RConnTagsString=__new0  BranchType=L  Resistance=1  Inductance=1E-7  SetiL0=off  InitialCurrent=0  Capacitance=1e-6  Setx0=off  InitialVoltage=0  Measurements=None
  Series RLC Branch7 : spsSeriesRLCBranchLib/Series RLC Branch  LConnTagsString=__new0  RConnTagsString=__new0  BranchType=RL  Resistance=0.6  Inductance=1e-6  SetiL0=off  InitialCurrent=0  Capacitance=1e-6  Setx0=off  InitialVoltage=0  Measurements=None
  Series RLC Branch9 : spsSeriesRLCBranchLib/Series RLC Branch  LConnTagsString=__new0  RConnTagsString=__new0  BranchType=L  Resistance=1  Inductance=0.4e-6  SetiL0=off  InitialCurrent=0  Capacitance=1e-6  Setx0=off  InitialVoltage=0  Measurements=None
  Terminator{,1..9} (10 alike) : Terminator
  Udc+ : PMIOPort  Side=Left
  udc- : PMIOPort  Port=2  Side=Left
  p1 : PMIOPort  Port=3  Side=Right
  p2 : PMIOPort  Port=4  Side=Right
  wires:
  Diode3/1 -> Terminator9/1
  IGBT3/1 -> Terminator5/1
  [n1] -> IGBT3/1
  IGBT1/1 -> Terminator4/1
  IGBT2/1 -> Terminator3/1
  IGBT/1 -> Terminator2/1
  [n2] -> IGBT1/1
  [p1] -> IGBT2/1
  Current Measurement1/1 -> Terminator/1
  Diode2/1 -> Terminator8/1
  [p2] -> IGBT/1
  Diode8/1 -> Terminator7/1
  Diode1/1 -> Terminator6/1
  Diode6/1 -> Terminator1/1
  Demux/3 -> [n2]
  PWM/1 -> Demux/1
  Demux/1 -> [p2]
  Demux/2 -> [p1]
  Demux/4 -> [n1]
  connections:
  Series RLC Branch10/LConn1 -- udc-/RConn1
  Series RLC Branch9/LConn1 -- Udc+/RConn1
  Diode6/RConn1 -- Series RLC Branch7/RConn1 -- Series RLC Branch2/LConn1
  Current Measurement1/LConn1 -- Series RLC Branch1/RConn1 -- Series RLC Branch3/LConn1 -- Series RLC Branch12/LConn1
  Diode3/LConn1 -- IGBT3/RConn1 -- Series RLC Branch14/RConn1
  Series RLC Branch3/RConn1 -- IGBT/LConn1 -- Diode8/RConn1
  Diode1/LConn1 -- Series RLC Branch5/RConn1 -- IGBT1/RConn1
  Current Measurement1/RConn1 -- Diode6/LConn1
  Diode2/RConn1 -- Series RLC Branch12/RConn1 -- IGBT2/LConn1
  p1/RConn1 -- Diode2/LConn1 -- Diode3/RConn1 -- IGBT3/LConn1 -- IGBT2/RConn1
  Series RLC Branch5/LConn1 -- Series RLC Branch14/LConn1 -- Series RLC Branch10/RConn1 -- Series RLC Branch2/RConn1
  Series RLC Branch1/LConn1 -- Series RLC Branch7/LConn1 -- Series RLC Branch9/RConn1
  p2/RConn1 -- IGBT1/LConn1 -- Diode1/RConn1 -- Diode8/LConn1 -- IGBT/RConn1

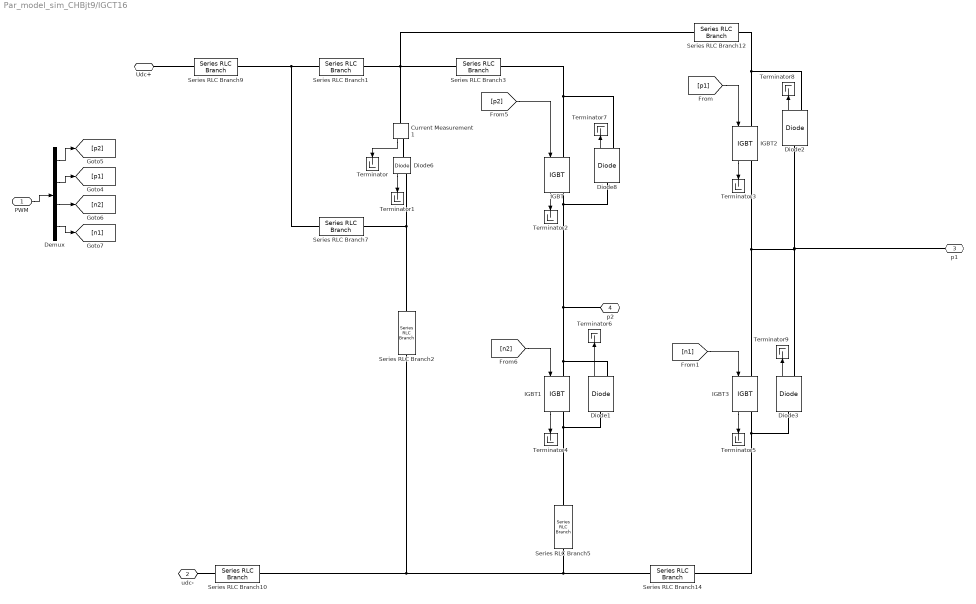
== system Par_model_sim_CHBjt9/IGCT16 ==
  PWM : Inport
  Current Measurement1 : spsCurrentMeasurementLib/Current Measurement  PhasorSimulation=off  OutputType=Complex  PSBequivalent=0
  Demux : Demux
  Diode{1..3,6,8} (5 alike) : spsDiodeLib/Diode  Ron=rto  Lon=0  Vf=vto  IC=0  UseSnubber=off  Rs=500  Cs=250e-9  Measurements=on
  IGBT{,1..3} (4 alike) : spsIGBTLib/IGBT  Ron=rt  Lon=0  Vf=vt  Tf=1e-6  Tt=2e-6  IC=0  Rs=1e5  Cs=inf  Measurements=on
  Series RLC Branch1 : spsSeriesRLCBranchLib/Series RLC Branch  LConnTagsString=__new0  RConnTagsString=__new0  BranchType=RL  Resistance=1e-5  Inductance=3.0E-6  SetiL0=off  InitialCurrent=0  Capacitance=1e-6  Setx0=off  InitialVoltage=0  Measurements=None
  Series RLC Branch10 : spsSeriesRLCBranchLib/Series RLC Branch  LConnTagsString=__new0  RConnTagsString=__new0  BranchType=L  Resistance=1  Inductance=0.4e-6  SetiL0=off  InitialCurrent=0  Capacitance=1e-6  Setx0=off  InitialVoltage=0  Measurements=None
  Series RLC Branch12 : spsSeriesRLCBranchLib/Series RLC Branch  LConnTagsString=__new0  RConnTagsString=__new0  BranchType=RL  Resistance=1e-5  Inductance=1E-9  SetiL0=off  InitialCurrent=0  Capacitance=1e-6  Setx0=off  InitialVoltage=0  Measurements=None
  Series RLC Branch14 : spsSeriesRLCBranchLib/Series RLC Branch  LConnTagsString=__new0  RConnTagsString=__new0  BranchType=L  Resistance=1  Inductance=1E-7  SetiL0=off  InitialCurrent=0  Capacitance=1e-6  Setx0=off  InitialVoltage=0  Measurements=None
  Series RLC Branch2 : spsSeriesRLCBranchLib/Series RLC Branch  LConnTagsString=__new0  RConnTagsString=__new0  BranchType=RC  Resistance=1e-5  Inductance=20e-6  SetiL0=off  InitialCurrent=0  Capacitance=17e-6  Setx0=off  InitialVoltage=0  Measurements=None
  Series RLC Branch3 : spsSeriesRLCBranchLib/Series RLC Branch  LConnTagsString=__new0  RConnTagsString=__new0  BranchType=RL  Resistance=1e-5  Inductance=1E-9  SetiL0=off  InitialCurrent=0  Capacitance=1e-6  Setx0=off  InitialVoltage=0  Measurements=None
  Series RLC Branch5 : spsSeriesRLCBranchLib/Series RLC Branch  LConnTagsString=__new0  RConnTagsString=__new0  BranchType=L  Resistance=1  Inductance=1E-7  SetiL0=off  InitialCurrent=0  Capacitance=1e-6  Setx0=off  InitialVoltage=0  Measurements=None
  Series RLC Branch7 : spsSeriesRLCBranchLib/Series RLC Branch  LConnTagsString=__new0  RConnTagsString=__new0  BranchType=RL  Resistance=0.6  Inductance=1e-6  SetiL0=off  InitialCurrent=0  Capacitance=1e-6  Setx0=off  InitialVoltage=0  Measurements=None
  Series RLC Branch9 : spsSeriesRLCBranchLib/Series RLC Branch  LConnTagsString=__new0  RConnTagsString=__new0  BranchType=L  Resistance=1  Inductance=0.4e-6  SetiL0=off  InitialCurrent=0  Capacitance=1e-6  Setx0=off  InitialVoltage=0  Measurements=None
  Terminator{,1..9} (10 alike) : Terminator
  Udc+ : PMIOPort  Side=Left
  udc- : PMIOPort  Port=2  Side=Left
  p1 : PMIOPort  Port=3  Side=Right
  p2 : PMIOPort  Port=4  Side=Right
  wires:
  Diode3/1 -> Terminator9/1
  IGBT3/1 -> Terminator5/1
  [n1] -> IGBT3/1
  IGBT1/1 -> Terminator4/1
  IGBT2/1 -> Terminator3/1
  IGBT/1 -> Terminator2/1
  [n2] -> IGBT1/1
  [p1] -> IGBT2/1
  Current Measurement1/1 -> Terminator/1
  Diode2/1 -> Terminator8/1
  [p2] -> IGBT/1
  Diode8/1 -> Terminator7/1
  Diode1/1 -> Terminator6/1
  Diode6/1 -> Terminator1/1
  Demux/3 -> [n2]
  PWM/1 -> Demux/1
  Demux/1 -> [p2]
  Demux/2 -> [p1]
  Demux/4 -> [n1]
  connections:
  Series RLC Branch10/LConn1 -- udc-/RConn1
  Series RLC Branch9/LConn1 -- Udc+/RConn1
  Diode6/RConn1 -- Series RLC Branch7/RConn1 -- Series RLC Branch2/LConn1
  Current Measurement1/LConn1 -- Series RLC Branch1/RConn1 -- Series RLC Branch3/LConn1 -- Series RLC Branch12/LConn1
  Diode3/LConn1 -- IGBT3/RConn1 -- Series RLC Branch14/RConn1
  Series RLC Branch3/RConn1 -- IGBT/LConn1 -- Diode8/RConn1
  Diode1/LConn1 -- Series RLC Branch5/RConn1 -- IGBT1/RConn1
  Current Measurement1/RConn1 -- Diode6/LConn1
  Diode2/RConn1 -- Series RLC Branch12/RConn1 -- IGBT2/LConn1
  p1/RConn1 -- Diode2/LConn1 -- Diode3/RConn1 -- IGBT3/LConn1 -- IGBT2/RConn1
  Series RLC Branch5/LConn1 -- Series RLC Branch14/LConn1 -- Series RLC Branch10/RConn1 -- Series RLC Branch2/RConn1
  Series RLC Branch1/LConn1 -- Series RLC Branch7/LConn1 -- Series RLC Branch9/RConn1
  p2/RConn1 -- IGBT1/LConn1 -- Diode1/RConn1 -- Diode8/LConn1 -- IGBT/RConn1
